simulink model "Bicycle_SCC_LKS"  (R2017a)
settings: Solver=ode45  StartTime=0.0  StopTime=30  MaxStep=0.001  RelTol=1e-3  EnableMultiTasking=on
PreLoadFcn:
  | load('Matrix.mat')
  | 
  | X0 = 25;         % 초기 X좌표 [m]
  | Y0 = 0;      % 초기 Y좌표 [m]
  | psi0 = 0;             % 초기 각도 [rad]
  | Vx0 = 100;           % 초기 속도 [km/h]
  | tf = 30;                 % 시뮬레이션 시간 [s]
  | 
  | % 제어기 설정 %
  | Q1 = 5;
  | Q2 = 3;
  | R =  2500;
  | PL = [-50-50i,-50+50i,-30,-20];
  | 
  | [K,L] = sfGain(Q1,Q2,R,PL);
model workspace (MAT data in the model file):
  Cf = 53220
  Cr = 39017
  Fx_Data = [-2029.26  -4058.51  -6087.76  -8117.01  -10146.3; -2029.26  -4058.51  -6087.76  -8117.01  -10146.3; -2053.55  -4107.12  -6160.67  -8214.24  -10267.8; -2084.58  -4169.16  -6253.75  -8338.33  -10422.9; -2125.47  -4250.95  -6376.42  -8501.91  -10627.4; -2181.64  -4363.28  -6544.93  -8726.56  -10908.2; -2262.94  -4525.87  -6788.82  -9051.76  -11314.7; -2388.22  -4776.46  -7164.69  -9552.92  -11941.1; -2476.95  -4953.9  -7430.85  -9907.79  -12384.7; -2586.89  -5173.78  -7760.68  -10347.6  -12934.4; -2634.75  -5269.5  -7904.24  -10539  -13173.7; -2680.7  -5361.4  -8042.1  -10722.8  -13403.5; -2717.36  -5434.73  -8152.09  -10869.4  -13586.8; -2729.82  -5459.63  -8189.45  -10919.3  -13649.1; -2689.78  -5379.54  -8069.32  -10759.1  -13448.8; -2548.95  -5097.92  -7646.88  -10195.8  -12744.8; -2240.07  -4480.13  -6720.21  -8960.27  -11200.3; -1701.43  -3402.86  -5104.29  -6805.72  -8507.15; -926.741  -1853.48  -2780.22  -3706.97  -4633.7; 0  0  0  0  0; 926.741  1853.48  2780.22  3706.97  4633.7; 1701.43  3402.86  5104.29  6805.72  8507.15; 2240.07  4480.13  6720.21  8960.27  11200.3; 2548.95  5097.92  7646.88  10195.8  12744.8; 2689.78  5379.54  8069.32  10759.1  13448.8; 2729.82  5459.63  8189.45  10919.3  13649.1; 2717.36  5434.73  8152.09  10869.4  13586.8; 2680.7  5361.4  8042.1  10722.8  13403.5; 2634.75  5269.5  7904.24  10539  13173.7; 2586.89  5173.78  7760.68  10347.6  12934.4; 2476.95  4953.9  7430.85  9907.79  12384.7; 2388.22  4776.46  7164.69  9552.92  11941.1; 2262.94  4525.87  6788.82  9051.76  11314.7; 2181.64  4363.28  6544.93  8726.56  10908.2; 2125.47  4250.95  6376.42  8501.91  10627.4; 2084.58  4169.16  6253.75  8338.33  10422.9; 2053.55  4107.12  6160.67  8214.24  10267.8; 2029.26  4058.51  6087.76  8117.01  10146.3; 2029.26  4058.51  6087.76  8117.01  10146.3]
  Fx_SL = [-1; -0.9; -0.8; -0.7; -0.6; -0.5; -0.4; -0.3; -0.25; -0.2; -0.18; -0.16; -0.14; -0.12; -0.1; -0.08; -0.06; -0.04; -0.02; 0; 0.02; 0.04; 0.06; 0.08; 0.1; 0.12; 0.14; 0.16; 0.18; 0.2; 0.25; 0.3; 0.4; 0.5; 0.6; 0.7; 0.8; 0.9; 1]
  Fx_W = [2105 3995 6120 7900 10100]
  Fy_Angle = [-20; -16; -14; -12; -10; -9.5; -9; -8.5; -8; -7.5; -7; -6.5; -6; -5.5; -5; -4.5; -4; -3.5; -3; -2.5; -2; -1.5; -1; -0.5; 0; 0.5; 1; 1.5; 2; 2.5; 3; 3.5; 4; 4.5; 5; 5.5; 6; 6.5; 7; 7.5; 8; 8.5; 9; 9.5; 10; 12; 14; 16; 18; 20]
  Fy_Data = [-1523.64 -1531.91 -1546.58 -1574.53 -1631.62 -1653.27 -1678.67 -1707.8 -1740.18 -1775.12 -1810.95 -1845.3 ... (250 elements, 50x5)]
  Fy_W = [1725 3500 6100 6950 9005]
  GearRatio = 17.25
  Iyy_Tire = 0.9
  Izz = 4192
  Pb2Tq_f = 300
  Pb2Tq_r = 150
  R_Tire = 0.33
  g = 9.81
  lf = 1.11
  lr = 1.6662
  m = 1530
  t2e = 2000
values from neighbouring files (symbols this model uses):
  P = polyfit(X*Scale,Y*Scale,4)    [Path_plot.m]
undefined symbols (not defined in the file or in its folder): A, B, K, L, sigbuilder_block
libraries: simulink x3
settings Model: Creator=Park  LastModifiedBy=edward
settings DataIOCC: SaveFormat=Array  SignalLoggingSaveFormat=ModelDataLogs
settings OptimizationCC: ExpressionDepthLimit=2147483647  LifeSpan=inf
settings DebuggingCC: UnderspecifiedInitializationDetection=Classic  MergeDetectMultiDrivingBlocksExec=none  SolverPrmCheckMsg=warning  MultiTaskDSMMsg=warning  MultiTaskCondExecSysMsg=none  FcnCallInpInsideContextMsg=warning  StateNameClashWarn=warning  StrictBusMsg=None  SFUnexpectedBacktrackingDiag=warning  SFNoUnconditionalDefaultTransitionDiag=warning  SFExecutionAtInitializationDiag=none
settings HardwareCC: ProdBitPerPointer=32  ProdBitPerSizeT=32  ProdBitPerPtrDiffT=32  ProdLargestAtomicFloat=None  ProdIntDivRoundTo=Undefined  ProdEndianess=Unspecified  ProdWordSize=32  ProdHWDeviceType=32-bit Generic
settings ModelReferenceCC: PropagateSignalLabelsOutOfModel=off
settings GRTTargetCC: TargetLangStandard=C89/C90 (ANSI)  GeneratePreprocessorConditionals=Disable all  CombineOutputUpdateFcns=off  GRTInterface=on
settings ConfigComp: CovMetricSettings=dw  CovHtmlReporting=on  CovSaveCumulativeToWorkspaceVar=on  CovSaveSingleToWorkspaceVar=on  CovExternalEMLEnable=off

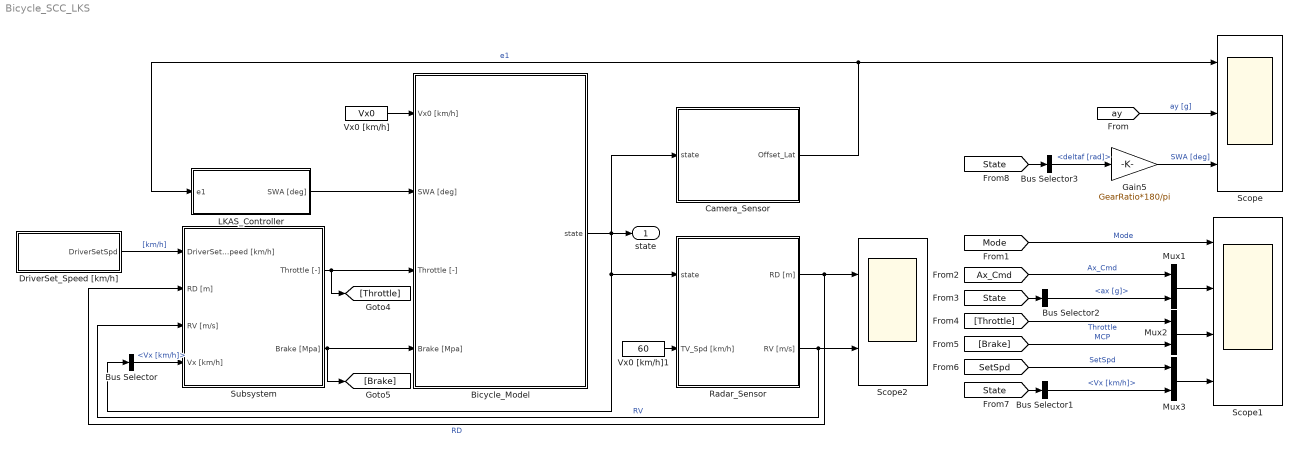
== system Bicycle_SCC_LKS ==
  Bicycle_Model : Subsystem
  Bus Selector : BusSelector  OutputSignals=Vx [km/h]
  Bus Selector1 : BusSelector  OutputSignals=Vx [km/h]
  Bus Selector2 : BusSelector  OutputSignals=ax [g]
  Bus Selector3 : BusSelector  OutputSignals=deltaf [rad]
  Camera_Sensor : Subsystem  TreatAsAtomicUnit=on  SystemSampleTime=1/100
  DriverSet_Speed [km/h] : Subsystem  Tag=STV Subsys  LoadFcn=sigbuilder_block('load');  StartFcn=sigbuilder_block('start');  StopFcn=sigbuilder_block('stop');  ClipboardFcn=sigbuilder_block('clipboard');  mask(Sigbuilder block){tuvar=[0:10]}
      mask help: Simulink:masks:SigbuilderBlock_MD
      mask init:
      | if ~strcmp(get_param(bdroot(gcbh),'SimulationStatus'),'stopped') tuvar = sigbuilder_block('maskInit'); end
      settings: CopyFcn=sigbuilder_block('copy');  DeleteFcn=sigbuilder_block('delete');  ModelCloseFcn=sigbuilder_block('modelClose');  PreSaveFcn=sigbuilder_block('preSave');  PauseFcn=sigbuilder_block('pause');  ContinueFcn=sigbuilder_block('continue');  NameChangeFcn=sigbuilder_block('namechange');  OpenFcn=sigbuilder_block('open',[6 36 708 710.25 ]);  CloseFcn=sigbuilder_block('close');
      mask Display: plot(0, 0, 100, 100,[2, 2, 32, 32, 2], [68, 8, 8, 68, 68],[32, 2], [38, 38], [32, 19, 2],[53, 60, 44], [32, 17, 17, 2],[16, 16, 31, 31]);txt = getActiveGroup(gcbh);text(2, 100, txt,'verticalAlignment', 'top');
  Gain5 : Gain  Gain=GearRatio*180/pi
  LKAS_Controller : Subsystem
  Mux1 : Mux  Inputs=2
  Mux2 : Mux  Inputs=2
  Mux3 : Mux  Inputs=2
  Radar_Sensor : Subsystem  SystemSampleTime=1/100
  Scope : Scope  NumInputPorts=3
  Scope1 : Scope  NumInputPorts=4
  Scope2 : Scope  NumInputPorts=2
  Subsystem : Subsystem
  Vx0 [km/h] : Constant  Value=Vx0
  Vx0 [km/h]1 : Constant  Value=60
  state : Outport
  wires:
  Vx0 [km/h]/1 -> Bicycle_Model/1(Vx0 [km/h])
  [ay] -> Scope/2  "ay [g]"
  Gain5/1 -> Scope/3  "SWA [deg]"
  DriverSet_Speed [km/h]/1(DriverSetSpd) -> Subsystem/1(DriverSet_Speed [km/h])  "[km/h]"
  [Mode] -> Scope1/1  "Mode"
  Mux1/1 -> Scope1/2
  [Ax_Cmd] -> Mux1/1  "Ax_Cmd"
  [State] -> Bus Selector2/1
  Mux2/1 -> Scope1/3
  [Brake] -> Mux2/2  "MCP"
  [Throttle] -> Mux2/1  "Throttle"
  Mux3/1 -> Scope1/4
  [SetSpd] -> Mux3/1  "SetSpd"
  LKAS_Controller/1(SWA [deg]) -> Bicycle_Model/2(SWA [deg])
  Bicycle_Model/1(state) -> Camera_Sensor/1(state), state/1, Radar_Sensor/1(state), Bus Selector/1
  Camera_Sensor/1(Offset_Lat) -> LKAS_Controller/1(e1), Scope/1  "e1"
  Subsystem/2(Brake [Mpa]) -> [Brake], Bicycle_Model/4(Brake [Mpa])
  Subsystem/1(Throttle [-]) -> Bicycle_Model/3(Throttle [-]), [Throttle]
  Bus Selector/1 -> Subsystem/4(Vx [km/h])  "<Vx [km/h]>"
  Radar_Sensor/1(RD [m]) -> Scope2/1, Subsystem/2(RD [m])  "RD"
  Radar_Sensor/2(RV [m/s]) -> Subsystem/3(RV [m/s]), Scope2/2  "RV"
  Vx0 [km/h]1/1 -> Radar_Sensor/2(TV_Spd [km/h])
  [State] -> Bus Selector1/1
  Bus Selector1/1 -> Mux3/2  "<Vx [km/h]>"
  Bus Selector2/1 -> Mux1/2  "<ax [g]>"
  [State] -> Bus Selector3/1
  Bus Selector3/1 -> Gain5/1  "<deltaf [rad]>"

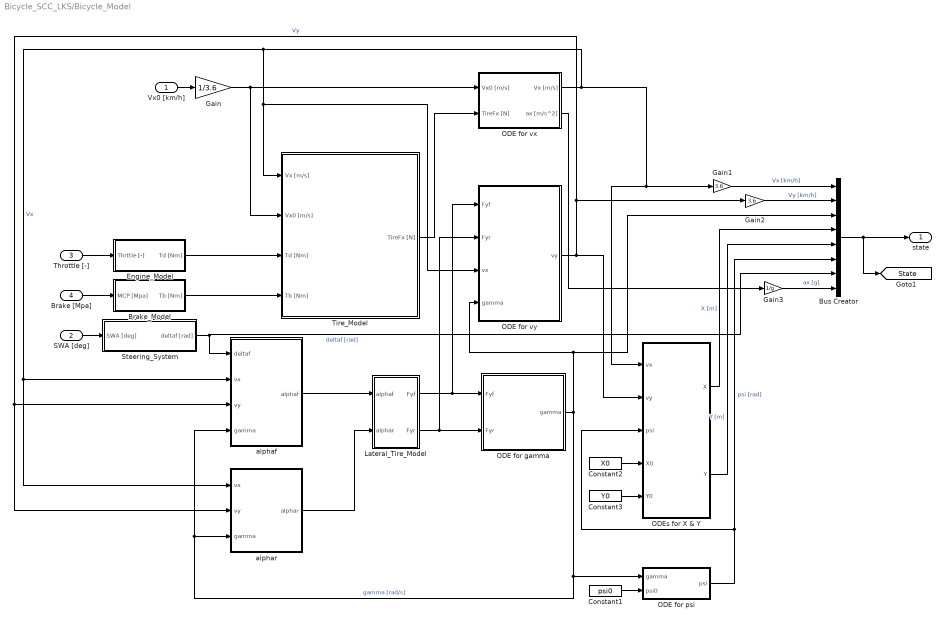
== system Bicycle_SCC_LKS/Bicycle_Model ==
  Vx0 [km/h] : Inport
  SWA [deg] : Inport  Port=2
  Throttle [-] : Inport  Port=3
  Brake [Mpa] : Inport  Port=4
  Brake_Model : Subsystem
  Bus Creator : BusCreator  Inputs=8
  Constant1 : Constant  Value=psi0
  Constant2 : Constant  Value=X0
  Constant3 : Constant  Value=Y0
  Engine_Model : Subsystem
  Gain : Gain  Gain=1/3.6
  Gain1 : Gain  Gain=3.6
  Gain2 : Gain  Gain=3.6
  Gain3 : Gain  Gain=1/g
  Lateral_Tire_Model : Subsystem
  ODE for gamma : Subsystem
  ODE for psi : Subsystem
  ODE for vx : Subsystem
  ODE for vy : Subsystem
  ODEs for X & Y : Subsystem
  Steering_System : Subsystem
  Tire_Model : Subsystem
  alphaf : Subsystem
  alphar : Subsystem
  state : Outport
  tag scope: State=global
  wires:
  alphaf/1(alphaf) -> Lateral_Tire_Model/1(alphaf)
  alphar/1(alphar) -> Lateral_Tire_Model/2(alphar)
  Lateral_Tire_Model/1(Fyf) -> ODE for vy/1(Fyf), ODE for gamma/1(Fyf)
  Lateral_Tire_Model/2(Fyr) -> ODE for vy/2(Fyr), ODE for gamma/2(Fyr)
  Bus Creator/1 -> [State], state/1
  Vx0 [km/h]/1 -> Gain/1
  Constant1/1 -> ODE for psi/2(psi0)
  SWA [deg]/1 -> Steering_System/1(SWA [deg])
  Constant2/1 -> ODEs for X & Y/4(X0)
  Constant3/1 -> ODEs for X & Y/5(Y0)
  ODE for psi/1(psi) -> ODEs for X & Y/3(psi), Bus Creator/6  "psi [rad]"
  ODEs for X & Y/1(X) -> Bus Creator/4  "X [m]"
  ODEs for X & Y/2(Y) -> Bus Creator/5  "Y [m]"
  Gain/1 -> ODE for vx/1(Vx0 [m/s]), Tire_Model/2(Vx0 [m/s])
  Engine_Model/1(Td [Nm]) -> Tire_Model/3(Td [Nm])
  Brake_Model/1(Tb [Nm]) -> Tire_Model/4(Tb [Nm])
  Brake [Mpa]/1 -> Brake_Model/1(MCP [Mpa])
  Throttle [-]/1 -> Engine_Model/1(Thrttle [-])
  Steering_System/1(deltaf [rad]) -> alphaf/1(deltaf), Bus Creator/7  "deltaf [rad]"
  ODE for vx/1(Vx [m/s]) -> alphaf/2(vx), alphar/1(vx), ODE for vy/3(vx), Tire_Model/1(Vx [m/s]), ODEs for X & Y/1(vx), Gain1/1  "Vx"
  ODE for gamma/1(gamma) -> Bus Creator/3, ODE for vy/4(gamma), ODE for psi/1(gamma), alphar/3(gamma), alphaf/4(gamma)  "gamma [rad/s]"
  Tire_Model/1(TireFx [N]) -> ODE for vx/2(TireFx [N])
  ODE for vx/2(ax [m/s^2]) -> Gain3/1
  ODE for vy/1(vy) -> alphar/2(vy), alphaf/3(vy), Gain2/1, ODEs for X & Y/2(vy)  "Vy"
  Gain1/1 -> Bus Creator/1  "Vx [km/h]"
  Gain2/1 -> Bus Creator/2  "Vy [km/h]"
  Gain3/1 -> Bus Creator/8  "ax [g]"

== system Bicycle_SCC_LKS/Camera_Sensor ==
  state : Inport
  Bus Selector : BusSelector  OutputSignals=X [m],Y [m],psi [rad]
  Compare To Constant : simulink/Logic and Bit Operations/Compare To Constant  relop=>=  const=350  OutDataTypeStr=boolean
  Gain : Gain  Gain=-1
  Level-2 MATLAB S-Function : M-S-Function  FunctionName=Error_Calculator_sfun
  Polynomial Coeff : Constant  Value=P
  Stop Simulation : Stop
  Terminator : Terminator
  Offset_Lat : Outport
  wires:
  state/1 -> Bus Selector/1
  Bus Selector/3 -> Level-2 MATLAB S-Function/4  "<psi [rad]>"
  Bus Selector/2 -> Level-2 MATLAB S-Function/3  "<Y [m]>"
  Bus Selector/1 -> Compare To Constant/1, Level-2 MATLAB S-Function/2  "<X [m]>"
  Level-2 MATLAB S-Function/1 -> Gain/1
  Polynomial Coeff/1 -> Level-2 MATLAB S-Function/1
  Level-2 MATLAB S-Function/2 -> Terminator/1
  Gain/1 -> Offset_Lat/1
  Compare To Constant/1 -> Stop Simulation/1

== system Bicycle_SCC_LKS/DriverSet_Speed [km//h] ==
  Demux : Demux  Tag=STV Demux  Outputs=1
  FromWs : FromWorkspace  Tag=STV FromWs  VariableName=tuvar  SampleTime=0
      SigBuilderData=|
      | common.afterFinalStr = 'Extrapolate'
      | common.sampleTime = 0
      | dataSet.timeRange = [0 30]
      | dataSet.name = 'Group 1'
      | sbobj.Groups.Name = 'Group 1'
      | sbobj.Groups.Signals.Name = 'DriverSetSpd'
      | sbobj.Groups.Signals.XData = [0 10 10 22 22 30]
      | sbobj.Groups.Signals.YData = [75 75 80 80 60 60]
      | sbobj.Groups.TimeRange = [0 30]
  DriverSetSpd : Outport  Tag=STV Outport
  wires:
  FromWs/1 -> Demux/1
  Demux/1 -> DriverSetSpd/1

== system Bicycle_SCC_LKS/LKAS_Controller ==
  e1 : Inport
  Ctrl_Law : Subsystem
  Observer : Subsystem
  Sum : Sum  Inputs=-+|
  SWA [deg] : Outport
  wires:
  Ctrl_Law/1(SWA [deg]) -> SWA [deg]/1, Observer/2(SWA [deg])
  Observer/1(e1_hat) -> Sum/1
  e1/1 -> Sum/2, Ctrl_Law/1(e1)
  Observer/2(e_hat) -> Ctrl_Law/2(e_hat)
  Sum/1 -> Observer/1(y_tilda)

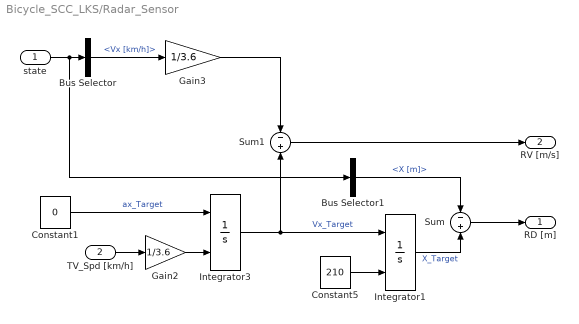
== system Bicycle_SCC_LKS/Radar_Sensor ==
  state : Inport
  TV_Spd [km/h] : Inport  Port=2
  Bus Selector : BusSelector  OutputSignals=Vx [km/h]
  Bus Selector1 : BusSelector  OutputSignals=X [m]
  Constant1 : Constant  Value=0
  Constant5 : Constant  Value=210
  Gain2 : Gain  Gain=1/3.6
  Gain3 : Gain  Gain=1/3.6
  Integrator1 : Integrator  InitialConditionSource=external  InitialCondition=500
  Integrator3 : Integrator  InitialConditionSource=external  InitialCondition=80  LimitOutput=on  LowerSaturationLimit=0
  Sum : Sum  Inputs=-+
  Sum1 : Sum  Inputs=-+
  RD [m] : Outport
  RV [m/s] : Outport  Port=2
  wires:
  TV_Spd [km/h]/1 -> Gain2/1
  Constant1/1 -> Integrator3/1  "ax_Target"
  Integrator3/1 -> Integrator1/1, Sum1/2  "Vx_Target"
  Integrator1/1 -> Sum/2  "X_Target"
  Constant5/1 -> Integrator1/2
  Sum/1 -> RD [m]/1
  Bus Selector1/1 -> Sum/1  "<X [m]>"
  Bus Selector/1 -> Gain3/1  "<Vx [km/h]>"
  Sum1/1 -> RV [m/s]/1
  Gain2/1 -> Integrator3/2
  Gain3/1 -> Sum1/1
  state/1 -> Bus Selector1/1, Bus Selector/1

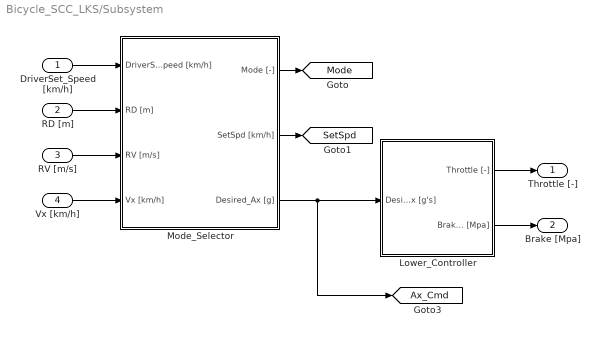
== system Bicycle_SCC_LKS/Subsystem ==
  DriverSet_Speed [km/h] : Inport
  RD [m] : Inport  Port=2
  RV [m/s] : Inport  Port=3
  Vx [km/h] : Inport  Port=4
  Lower_Controller : Subsystem
  Mode_Selector : Subsystem
  Throttle [-] : Outport
  Brake [Mpa] : Outport  Port=2
  tag scope: Ax_Cmd=global, Mode=global, SetSpd=global
  wires:
  Mode_Selector/3(Desired_Ax [g]) -> [Ax_Cmd], Lower_Controller/1(Desired_Ax [g's])
  Mode_Selector/1(Mode [-]) -> [Mode]
  Mode_Selector/2(SetSpd [km/h]) -> [SetSpd]
  RV [m/s]/1 -> Mode_Selector/3(RV [m/s])
  RD [m]/1 -> Mode_Selector/2(RD [m])
  DriverSet_Speed [km/h]/1 -> Mode_Selector/1(DriverSet_Speed [km/h])
  Vx [km/h]/1 -> Mode_Selector/4(Vx [km/h])
  Lower_Controller/1(Throttle [-]) -> Throttle [-]/1
  Lower_Controller/2(Brake [Mpa]) -> Brake [Mpa]/1

== system Bicycle_SCC_LKS/Bicycle_Model/Brake_Model ==
  MCP [Mpa] : Inport
  Gain : Gain  Gain=2*Pb2Tq_f
  Gain1 : Gain  Gain=2*Pb2Tq_r
  Mux : Mux  Inputs=2
  Transfer Fcn : TransferFcn  Denominator=[0.06 1]
  Transfer Fcn1 : TransferFcn  Denominator=[0.06 1]
  Tb [Nm] : Outport
  wires:
  Gain/1 -> Transfer Fcn/1  "Tb_f [Nm]"
  Gain1/1 -> Transfer Fcn1/1  "Tb_r [Nm]"
  MCP [Mpa]/1 -> Gain1/1, Gain/1
  Mux/1 -> Tb [Nm]/1
  Transfer Fcn/1 -> Mux/1
  Transfer Fcn1/1 -> Mux/2

== system Bicycle_SCC_LKS/Bicycle_Model/Engine_Model ==
  Thrttle [-] : Inport
  Gain : Gain  Gain=t2e
  Transfer Fcn : TransferFcn  Numerator=[100]  Denominator=[1 2*0.5*10 100]
  Td [Nm] : Outport
  wires:
  Thrttle [-]/1 -> Gain/1
  Gain/1 -> Transfer Fcn/1
  Transfer Fcn/1 -> Td [Nm]/1

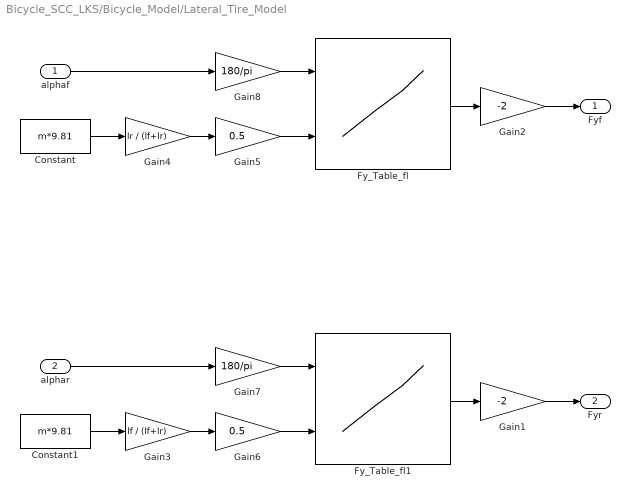
== system Bicycle_SCC_LKS/Bicycle_Model/Lateral_Tire_Model ==
  alphaf : Inport
  alphar : Inport  Port=2
  Constant : Constant  Value=m*9.81
  Constant1 : Constant  Value=m*9.81
  Fy_Table_fl : Lookup2D  RowIndex=Fy_Angle  ColumnIndex=Fy_W  Table=Fy_Data  LookUpMeth=Interpolation-Use End Values  SaturateOnIntegerOverflow=on
  Fy_Table_fl1 : Lookup2D  RowIndex=Fy_Angle  ColumnIndex=Fy_W  Table=Fy_Data  LookUpMeth=Interpolation-Use End Values  SaturateOnIntegerOverflow=on
  Gain1 : Gain  Gain=-2
  Gain2 : Gain  Gain=-2
  Gain3 : Gain  Gain=lf / (lf+lr)
  Gain4 : Gain  Gain=lr / (lf+lr)
  Gain5 : Gain  Gain=0.5
  Gain6 : Gain  Gain=0.5
  Gain7 : Gain  Gain=180/pi
  Gain8 : Gain  Gain=180/pi
  Fyf : Outport
  Fyr : Outport  Port=2
  wires:
  alphaf/1 -> Gain8/1
  Constant/1 -> Gain4/1
  Gain4/1 -> Gain5/1
  Gain5/1 -> Fy_Table_fl/2
  Fy_Table_fl/1 -> Gain2/1
  Gain2/1 -> Fyf/1
  Gain8/1 -> Fy_Table_fl/1
  alphar/1 -> Gain7/1
  Gain3/1 -> Gain6/1
  Gain6/1 -> Fy_Table_fl1/2
  Fy_Table_fl1/1 -> Gain1/1
  Gain7/1 -> Fy_Table_fl1/1
  Constant1/1 -> Gain3/1
  Gain1/1 -> Fyr/1

== system Bicycle_SCC_LKS/Bicycle_Model/ODE for gamma ==
  Fyf : Inport
  Fyr : Inport  Port=2
  Gain4 : Gain  Gain=1/Izz
  Gain5 : Gain  Gain=lf
  Gain6 : Gain  Gain=lr
  Integrator2 : Integrator
  Sum2 : Sum  Inputs=+-
  gamma : Outport
  wires:
  Sum2/1 -> Gain4/1
  Gain4/1 -> Integrator2/1
  Gain5/1 -> Sum2/1
  Gain6/1 -> Sum2/2
  Fyf/1 -> Gain5/1
  Integrator2/1 -> gamma/1  "gamma"
  Fyr/1 -> Gain6/1

== system Bicycle_SCC_LKS/Bicycle_Model/ODE for psi ==
  gamma : Inport
  psi0 : Inport  Port=2
  Integrator : Integrator  InitialConditionSource=external
  psi : Outport
  wires:
  gamma/1 -> Integrator/1  "dpsi"
  Integrator/1 -> psi/1
  psi0/1 -> Integrator/2

== system Bicycle_SCC_LKS/Bicycle_Model/ODE for vx ==
  Vx0 [m/s] : Inport
  TireFx [N] : Inport  Port=2
  Demux : Demux  Outputs=2
  Gain : Gain  Gain=1/m
  Integrator : Integrator  InitialConditionSource=external
  Sum : Sum
  Vx [m/s] : Outport
  ax [m/s^2] : Outport  Port=2
  wires:
  Vx0 [m/s]/1 -> Integrator/2
  Integrator/1 -> Vx [m/s]/1
  Sum/1 -> Gain/1
  Gain/1 -> Integrator/1, ax [m/s^2]/1
  TireFx [N]/1 -> Demux/1
  Demux/1 -> Sum/1
  Demux/2 -> Sum/2

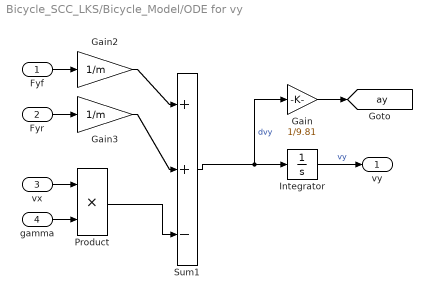
== system Bicycle_SCC_LKS/Bicycle_Model/ODE for vy ==
  Fyf : Inport
  Fyr : Inport  Port=2
  vx : Inport  Port=3
  gamma : Inport  Port=4
  Gain : Gain  Gain=1/9.81
  Gain2 : Gain  Gain=1/m
  Gain3 : Gain  Gain=1/m
  Integrator : Integrator
  Product : Product  RndMeth=Zero
  Sum1 : Sum  Inputs=++|-
  vy : Outport
  tag scope: ay=global
  wires:
  Gain2/1 -> Sum1/1
  Gain3/1 -> Sum1/2
  Sum1/1 -> Gain/1, Integrator/1  "dvy"
  Product/1 -> Sum1/3
  Fyf/1 -> Gain2/1
  Fyr/1 -> Gain3/1
  Integrator/1 -> vy/1  "vy"
  vx/1 -> Product/1
  gamma/1 -> Product/2
  Gain/1 -> [ay]

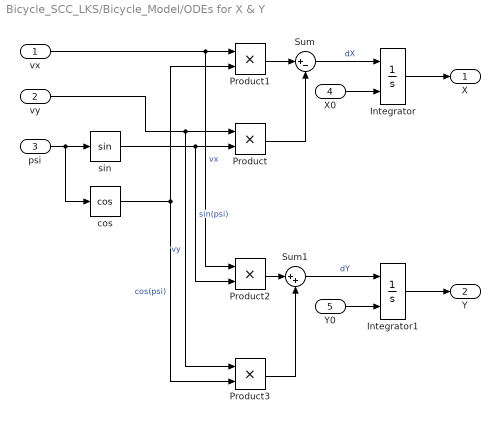
== system Bicycle_SCC_LKS/Bicycle_Model/ODEs for X & Y ==
  vx : Inport
  vy : Inport  Port=2
  psi : Inport  Port=3
  X0 : Inport  Port=4
  Y0 : Inport  Port=5
  Integrator : Integrator  InitialConditionSource=external  InitialCondition=42.14
  Integrator1 : Integrator  InitialConditionSource=external  InitialCondition=-0.3743
  Product{,1..3} (4 alike) : Product  RndMeth=Zero
  Sum : Sum  Inputs=|+-
  Sum1 : Sum  Inputs=|++
  cos : Trigonometry  Operator=cos
  sin : Trigonometry
  X : Outport
  Y : Outport  Port=2
  wires:
  psi/1 -> sin/1, cos/1
  sin/1 -> Product/2, Product2/2  "sin(psi)"
  vy/1 -> Product/1, Product3/1  "vy"
  vx/1 -> Product1/1, Product2/1  "vx"
  cos/1 -> Product1/2, Product3/2  "cos(psi)"
  Product1/1 -> Sum/1
  Product/1 -> Sum/2
  Sum/1 -> Integrator/1  "dX"
  Product2/1 -> Sum1/1
  Product3/1 -> Sum1/2
  Sum1/1 -> Integrator1/1  "dY"
  Integrator/1 -> X/1
  Integrator1/1 -> Y/1
  X0/1 -> Integrator/2
  Y0/1 -> Integrator1/2

== system Bicycle_SCC_LKS/Bicycle_Model/Steering_System ==
  SWA [deg] : Inport
  Gain : Gain  Gain=1/GearRatio
  Gain5 : Gain  Gain=pi/180
  Rate Limiter : RateLimiter  RisingSlewLimit=500  FallingSlewLimit=-500  SampleTimeMode=inherited
  Saturation : Saturate  UpperLimit=450  LowerLimit=-450
  deltaf [rad] : Outport
  wires:
  Gain/1 -> Gain5/1
  Gain5/1 -> deltaf [rad]/1
  SWA [deg]/1 -> Saturation/1
  Rate Limiter/1 -> Gain/1
  Saturation/1 -> Rate Limiter/1

== system Bicycle_SCC_LKS/Bicycle_Model/Tire_Model ==
  Vx [m/s] : Inport
  Vx0 [m/s] : Inport  Port=2
  Td [Nm] : Inport  Port=3
  Tb [Nm] : Inport  Port=4
  Long.Tire_Model : Subsystem
  ODE_for_Wss : Subsystem
  Slip_Ratio_Calculator : Subsystem
  TireFx [N] : Outport
  wires:
  Long.Tire_Model/1(TireFx [N]) -> TireFx [N]/1, ODE_for_Wss/1(TireFx [N])
  Slip_Ratio_Calculator/1(lamda [-]) -> Long.Tire_Model/1(lamda [-])
  Vx [m/s]/1 -> Slip_Ratio_Calculator/1(Vx [m/s])
  Vx0 [m/s]/1 -> ODE_for_Wss/2(Vx0 [m/s])
  Td [Nm]/1 -> ODE_for_Wss/3(Td [Nm])
  Tb [Nm]/1 -> ODE_for_Wss/4(Tb [Nm])
  ODE_for_Wss/1(Wss [rad/s]) -> Slip_Ratio_Calculator/2(Wss [rad/s])

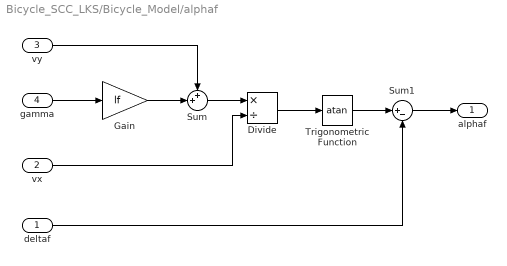
== system Bicycle_SCC_LKS/Bicycle_Model/alphaf ==
  deltaf : Inport
  vx : Inport  Port=2
  vy : Inport  Port=3
  gamma : Inport  Port=4
  Divide : Product  Inputs=*/
  Gain : Gain  Gain=lf
  Sum : Sum  Inputs=++|
  Sum1 : Sum  Inputs=|+-
  Trigonometric Function : Trigonometry  Operator=atan
  alphaf : Outport
  wires:
  gamma/1 -> Gain/1
  vy/1 -> Sum/1
  Gain/1 -> Sum/2
  Sum/1 -> Divide/1
  vx/1 -> Divide/2
  Divide/1 -> Trigonometric Function/1
  Trigonometric Function/1 -> Sum1/1
  deltaf/1 -> Sum1/2
  Sum1/1 -> alphaf/1

== system Bicycle_SCC_LKS/Bicycle_Model/alphar ==
  vx : Inport
  vy : Inport  Port=2
  gamma : Inport  Port=3
  Divide : Product  Inputs=*/
  Gain : Gain  Gain=lr
  Sum : Sum  Inputs=+-|
  Trigonometric Function : Trigonometry  Operator=atan
  alphar : Outport
  wires:
  Trigonometric Function/1 -> alphar/1
  Divide/1 -> Trigonometric Function/1
  vx/1 -> Divide/2
  Sum/1 -> Divide/1
  Gain/1 -> Sum/2
  vy/1 -> Sum/1
  gamma/1 -> Gain/1

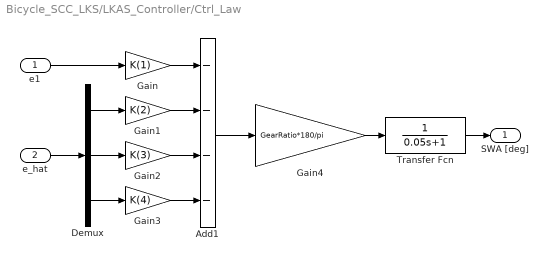
== system Bicycle_SCC_LKS/LKAS_Controller/Ctrl_Law ==
  e1 : Inport
  e_hat : Inport  Port=2
  Add1 : Sum  Inputs=----
  Demux : Demux  Outputs=3
  Gain : Gain  Gain=K(1)
  Gain1 : Gain  Gain=K(2)
  Gain2 : Gain  Gain=K(3)
  Gain3 : Gain  Gain=K(4)
  Gain4 : Gain  Gain=GearRatio*180/pi
  Transfer Fcn : TransferFcn  Denominator=[0.05 1]
  SWA [deg] : Outport
  wires:
  Gain3/1 -> Add1/4
  Gain2/1 -> Add1/3
  Gain1/1 -> Add1/2
  Demux/3 -> Gain3/1
  Demux/2 -> Gain2/1
  Demux/1 -> Gain1/1
  e1/1 -> Gain/1
  Gain/1 -> Add1/1
  e_hat/1 -> Demux/1
  Add1/1 -> Gain4/1
  Gain4/1 -> Transfer Fcn/1
  Transfer Fcn/1 -> SWA [deg]/1

== system Bicycle_SCC_LKS/LKAS_Controller/Observer ==
  y_tilda : Inport
  SWA [deg] : Inport  Port=2
  Demux : Demux
  Gain5 : Gain  Gain=1/GearRatio*pi/180
  Mux : Mux  Inputs=2
  Mux1 : Mux  Inputs=3
  State-Space : StateSpace  A=A  B=[B L']  C=diag([1 1 1 1])  D=zeros(4,2)  X0=0  ContinuousStateAttributes={'e1','e1_dot','e2','e2_dot'}
  e1_hat : Outport
  e_hat : Outport  Port=2
  wires:
  Mux/1 -> State-Space/1
  State-Space/1 -> Demux/1
  Demux/1 -> e1_hat/1  "e1_hat"
  y_tilda/1 -> Mux/2
  Demux/3 -> Mux1/2  "e2_hat"
  Demux/2 -> Mux1/1  "e1_dot_hat"
  Demux/4 -> Mux1/3  "e2_dot_hat"
  Mux1/1 -> e_hat/1
  SWA [deg]/1 -> Gain5/1
  Gain5/1 -> Mux/1

== system Bicycle_SCC_LKS/Subsystem/Lower_Controller ==
  Desired_Ax [g's] : Inport
  Brake_Controller : Subsystem  RequirementInfo={} %GIDa_b1ea8aed_7b1f_4164_abf5_d515769a3c42
  Throttle_Controller : Subsystem  RequirementInfo={} %GIDa_0f87ebad_d791_4b9c_99aa_9bea3fba617a
  Throttle [-] : Outport
  Brake [Mpa] : Outport  Port=2
  wires:
  Desired_Ax [g's]/1 -> Throttle_Controller/1(Ax_cmd [g's]), Brake_Controller/1(Ax_cmd [g's])
  Throttle_Controller/1(Throttle [-]) -> Throttle [-]/1
  Brake_Controller/1(Brake [Mpa]) -> Brake [Mpa]/1

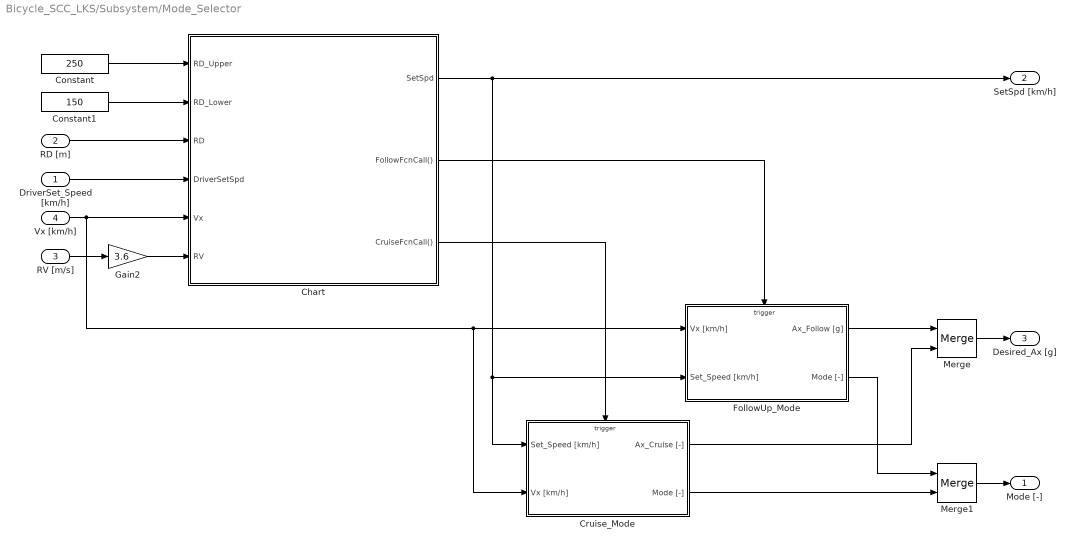
== system Bicycle_SCC_LKS/Subsystem/Mode_Selector ==
  DriverSet_Speed [km/h] : Inport
  RD [m] : Inport  Port=2
  RV [m/s] : Inport  Port=3
  Vx [km/h] : Inport  Port=4
  Chart : Stateflow chart  TreatAsAtomicUnit=on
  Constant : Constant  Value=250
  Constant1 : Constant  Value=150
  Cruise_Mode : Subsystem
  FollowUp_Mode : Subsystem
  Gain2 : Gain  Gain=3.6
  Merge : Merge
  Merge1 : Merge
  Mode [-] : Outport
  SetSpd [km/h] : Outport  Port=2
  Desired_Ax [g] : Outport  Port=3
  wires:
  Constant1/1 -> Chart/2(RD_Lower)
  Constant/1 -> Chart/1(RD_Upper)
  RV [m/s]/1 -> Gain2/1
  Cruise_Mode/2(Mode [-]) -> Merge1/2
  FollowUp_Mode/2(Mode [-]) -> Merge1/1
  Cruise_Mode/1(Ax_Cruise [-]) -> Merge/2
  FollowUp_Mode/1(Ax_Follow [g]) -> Merge/1
  Chart/1(SetSpd) -> SetSpd [km/h]/1, FollowUp_Mode/2(Set_Speed [km/h]), Cruise_Mode/1(Set_Speed [km/h])
  DriverSet_Speed [km/h]/1 -> Chart/4(DriverSetSpd)
  Chart/3(CruiseFcnCall()) -> Cruise_Mode/Trigger
  Chart/2(FollowFcnCall()) -> FollowUp_Mode/Trigger
  RD [m]/1 -> Chart/3(RD)
  Merge1/1 -> Mode [-]/1
  Merge/1 -> Desired_Ax [g]/1
  Vx [km/h]/1 -> Chart/5(Vx), Cruise_Mode/2(Vx [km/h]), FollowUp_Mode/1(Vx [km/h])
  Gain2/1 -> Chart/6(RV)

== system Bicycle_SCC_LKS/Bicycle_Model/Tire_Model/Long.Tire_Model ==
  lamda [-] : Inport
  Demux : Demux  Outputs=2
  Fx_f_Calculator : Subsystem
  Fx_r_Calculator : Subsystem
  Mux : Mux  Inputs=2
  TireFx [N] : Outport
  wires:
  lamda [-]/1 -> Demux/1
  Demux/1 -> Fx_f_Calculator/1(lamda_f [-])
  Demux/2 -> Fx_r_Calculator/1(lamda_r [-])
  Fx_f_Calculator/1(TireFx _f [N]) -> Mux/1
  Fx_r_Calculator/1(TireFx _r [N]) -> Mux/2
  Mux/1 -> TireFx [N]/1

== system Bicycle_SCC_LKS/Bicycle_Model/Tire_Model/ODE_for_Wss ==
  TireFx [N] : Inport
  Vx0 [m/s] : Inport  Port=2
  Td [Nm] : Inport  Port=3
  Tb [Nm] : Inport  Port=4
  Demux : Demux  Outputs=2
  Demux1 : Demux  Outputs=2
  Mux : Mux  Inputs=2
  ODE_for_Wss_f : Subsystem
  ODE_for_Wss_r : Subsystem
  Wss [rad/s] : Outport
  wires:
  Demux1/1 -> ODE_for_Wss_f/3(TireFx _f [N])  "TireFx _f [N]"
  Td [Nm]/1 -> ODE_for_Wss_f/1(Td_f [Nm])
  Vx0 [m/s]/1 -> ODE_for_Wss_r/1(Vx0 [m/s]), ODE_for_Wss_f/2(Vx0 [m/s])
  Tb [Nm]/1 -> Demux/1
  Demux/1 -> ODE_for_Wss_f/4(Tb_f [Nm])
  Demux/2 -> ODE_for_Wss_r/3(Tb_r [Nm])
  TireFx [N]/1 -> Demux1/1
  Demux1/2 -> ODE_for_Wss_r/2(TireFx _r [N])  "TireFx _r [N]"
  ODE_for_Wss_f/1(Wss_f [rad/s]) -> Mux/1
  ODE_for_Wss_r/1(Wss_r [rad/s]) -> Mux/2
  Mux/1 -> Wss [rad/s]/1

== system Bicycle_SCC_LKS/Bicycle_Model/Tire_Model/Slip_Ratio_Calculator ==
  Vx [m/s] : Inport
  Wss [rad/s] : Inport  Port=2
  Demux : Demux  Outputs=2
  Mux : Mux  Inputs=2
  lamda_f_Calculator : Subsystem
  lamda_r_Calculator1 : Subsystem
  lamda [-] : Outport
  wires:
  Vx [m/s]/1 -> lamda_f_Calculator/2(Vx [m/s]), lamda_r_Calculator1/2(Vx [m/s])
  lamda_f_Calculator/1(lamda_f [-]) -> Mux/1  "lamda_f [-]"
  lamda_r_Calculator1/1(lamda_r [-]) -> Mux/2  "lamda_r [-]"
  Mux/1 -> lamda [-]/1
  Wss [rad/s]/1 -> Demux/1
  Demux/1 -> lamda_f_Calculator/1(Wss_f [rad/s])  "Wss_f [rad/s]"
  Demux/2 -> lamda_r_Calculator1/1(Wss_r [rad/s])  "Wss_r [rad/s]"

== system Bicycle_SCC_LKS/Subsystem/Lower_Controller/Brake_Controller ==
  Ax_cmd [g's] : Inport
  Compare To Zero : simulink/Logic and Bit Operations/Compare To Zero  relop=<=  OutDataTypeStr=boolean
  Data Type Conversion : DataTypeConversion  OutDataTypeStr=double
  Gain : Gain  Gain=-1
  Gain1 : Gain  Gain=0.05
  Gain2 : Gain  Gain=12
  Integrator : Integrator  ExternalReset=rising
  Saturation : Saturate  UpperLimit=4  LowerLimit=0
  Sum : Sum
  Brake [Mpa] : Outport
  wires:
  Gain/1 -> Gain2/1, Gain1/1, Compare To Zero/1
  Saturation/1 -> Brake [Mpa]/1
  Sum/1 -> Saturation/1
  Ax_cmd [g's]/1 -> Gain/1
  Gain2/1 -> Sum/1
  Compare To Zero/1 -> Data Type Conversion/1
  Integrator/1 -> Sum/2
  Gain1/1 -> Integrator/1
  Data Type Conversion/1 -> Integrator/2

== system Bicycle_SCC_LKS/Subsystem/Lower_Controller/Throttle_Controller ==
  Ax_cmd [g's] : Inport
  Compare To Zero : simulink/Logic and Bit Operations/Compare To Zero  relop=<=  OutDataTypeStr=boolean
  Data Type Conversion : DataTypeConversion  OutDataTypeStr=double
  Gain1 : Gain  Gain=0.5
  Gain2 : Gain  Gain=7
  Integrator : Integrator  ExternalReset=rising
  Saturation : Saturate  UpperLimit=0.7  LowerLimit=0
  Sum : Sum
  Throttle [-] : Outport
  wires:
  Saturation/1 -> Throttle [-]/1
  Sum/1 -> Saturation/1
  Ax_cmd [g's]/1 -> Gain2/1, Gain1/1, Compare To Zero/1
  Gain2/1 -> Sum/1
  Compare To Zero/1 -> Data Type Conversion/1
  Integrator/1 -> Sum/2
  Gain1/1 -> Integrator/1
  Data Type Conversion/1 -> Integrator/2

== system Bicycle_SCC_LKS/Subsystem/Mode_Selector/Cruise_Mode ==
  Set_Speed [km/h] : Inport
  Vx [km/h] : Inport  Port=2
  function : TriggerPort  TriggerType=function-call  VariantControl=Variant
  Divide : Product  Inputs=/*
  Gain : Gain  Gain=1.2
  Mode1 : Constant  Value=0
  Saturation : Saturate  UpperLimit=0.3  LowerLimit=-0.3
  Sum : Sum  Inputs=|+-
  Ax_Cruise [-] : Outport
  Mode [-] : Outport  Port=2
  wires:
  Vx [km/h]/1 -> Sum/2
  Mode1/1 -> Mode [-]/1
  Saturation/1 -> Ax_Cruise [-]/1
  Divide/1 -> Gain/1  "Normalized_Vx"
  Sum/1 -> Divide/2
  Set_Speed [km/h]/1 -> Divide/1, Sum/1
  Gain/1 -> Saturation/1

== system Bicycle_SCC_LKS/Subsystem/Mode_Selector/FollowUp_Mode ==
  Vx [km/h] : Inport
  Set_Speed [km/h] : Inport  Port=2
  function : TriggerPort  TriggerType=function-call  VariantControl=Variant
  Divide : Product  Inputs=/*
  Gain : Gain  Gain=2
  Mode1 : Constant
  Saturation1 : Saturate  UpperLimit=0.4  LowerLimit=-0.4
  Sum1 : Sum  Inputs=|+-
  Ax_Follow [g] : Outport
  Mode [-] : Outport  Port=2
  wires:
  Vx [km/h]/1 -> Sum1/2
  Set_Speed [km/h]/1 -> Sum1/1, Divide/1
  Saturation1/1 -> Ax_Follow [g]/1
  Divide/1 -> Gain/1  "Normalized_Vx"
  Sum1/1 -> Divide/2
  Mode1/1 -> Mode [-]/1
  Gain/1 -> Saturation1/1

== system Bicycle_SCC_LKS/Bicycle_Model/Tire_Model/Long.Tire_Model/Fx_f_Calculator ==
  lamda_f [-] : Inport
  Constant : Constant  Value=m*9.81
  Fx_Table_fl : Lookup2D  RowIndex=Fx_SL  ColumnIndex=Fx_W  Table=Fx_Data  SaturateOnIntegerOverflow=on
  Gain : Gain  Gain=lr / (lf+lr)
  Gain1 : Gain  Gain=2
  Gain4 : Gain  Gain=0.5
  TireFx _f [N] : Outport
  wires:
  Gain1/1 -> TireFx _f [N]/1
  lamda_f [-]/1 -> Fx_Table_fl/1
  Constant/1 -> Gain/1
  Gain/1 -> Gain4/1
  Gain4/1 -> Fx_Table_fl/2  "Wf [N]"
  Fx_Table_fl/1 -> Gain1/1

== system Bicycle_SCC_LKS/Bicycle_Model/Tire_Model/Long.Tire_Model/Fx_r_Calculator ==
  lamda_r [-] : Inport
  Constant1 : Constant  Value=m*9.81
  Fx_Table_fl1 : Lookup2D  RowIndex=Fx_SL  ColumnIndex=Fx_W  Table=Fx_Data  SaturateOnIntegerOverflow=on
  Gain2 : Gain  Gain=lf / (lf+lr)
  Gain3 : Gain  Gain=2
  Gain5 : Gain  Gain=0.5
  TireFx _r [N] : Outport
  wires:
  lamda_r [-]/1 -> Fx_Table_fl1/1
  Constant1/1 -> Gain2/1
  Fx_Table_fl1/1 -> Gain3/1
  Gain2/1 -> Gain5/1
  Gain5/1 -> Fx_Table_fl1/2  "Wr [N]"
  Gain3/1 -> TireFx _r [N]/1

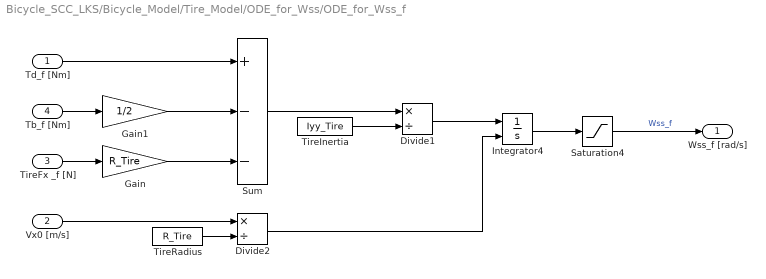
== system Bicycle_SCC_LKS/Bicycle_Model/Tire_Model/ODE_for_Wss/ODE_for_Wss_f ==
  Td_f [Nm] : Inport
  Vx0 [m/s] : Inport  Port=2
  TireFx _f [N] : Inport  Port=3
  Tb_f [Nm] : Inport  Port=4
  Divide1 : Product  Inputs=*/
  Divide2 : Product  Inputs=*/
  Gain : Gain  Gain=R_Tire
  Gain1 : Gain  Gain=1/2
  Integrator4 : Integrator  InitialConditionSource=external
  Saturation4 : Saturate  UpperLimit=255  LowerLimit=0
  Sum : Sum  Inputs=+--
  TireInertia : Constant  Value=Iyy_Tire
  TireRadius : Constant  Value=R_Tire
  Wss_f [rad/s] : Outport
  wires:
  Gain/1 -> Sum/3
  Td_f [Nm]/1 -> Sum/1
  Tb_f [Nm]/1 -> Gain1/1
  TireFx _f [N]/1 -> Gain/1
  Sum/1 -> Divide1/1
  TireInertia/1 -> Divide1/2
  Divide1/1 -> Integrator4/1
  TireRadius/1 -> Divide2/2
  Vx0 [m/s]/1 -> Divide2/1
  Divide2/1 -> Integrator4/2
  Integrator4/1 -> Saturation4/1
  Saturation4/1 -> Wss_f [rad/s]/1  "Wss_f"
  Gain1/1 -> Sum/2

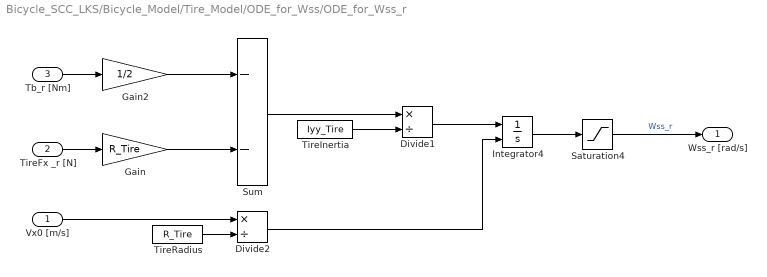
== system Bicycle_SCC_LKS/Bicycle_Model/Tire_Model/ODE_for_Wss/ODE_for_Wss_r ==
  Vx0 [m/s] : Inport
  TireFx _r [N] : Inport  Port=2
  Tb_r [Nm] : Inport  Port=3
  Divide1 : Product  Inputs=*/
  Divide2 : Product  Inputs=*/
  Gain : Gain  Gain=R_Tire
  Gain2 : Gain  Gain=1/2
  Integrator4 : Integrator  InitialConditionSource=external
  Saturation4 : Saturate  UpperLimit=255  LowerLimit=0
  Sum : Sum  Inputs=--
  TireInertia : Constant  Value=Iyy_Tire
  TireRadius : Constant  Value=R_Tire
  Wss_r [rad/s] : Outport
  wires:
  Saturation4/1 -> Wss_r [rad/s]/1  "Wss_r"
  Integrator4/1 -> Saturation4/1
  Divide2/1 -> Integrator4/2
  Vx0 [m/s]/1 -> Divide2/1
  TireRadius/1 -> Divide2/2
  Divide1/1 -> Integrator4/1
  TireInertia/1 -> Divide1/2
  Sum/1 -> Divide1/1
  TireFx _r [N]/1 -> Gain/1
  Tb_r [Nm]/1 -> Gain2/1
  Gain/1 -> Sum/2
  Gain2/1 -> Sum/1

== system Bicycle_SCC_LKS/Bicycle_Model/Tire_Model/Slip_Ratio_Calculator/lamda_f_Calculator ==
  Wss_f [rad/s] : Inport
  Vx [m/s] : Inport  Port=2
  Divide : Product  Inputs=*/
  Product2 : Product  RndMeth=Zero
  Saturation4 : Saturate  UpperLimit=1  LowerLimit=-1
  Subtract : Sum  Inputs=-+
  TireRadius : Constant  Value=R_Tire
  lamda_f [-] : Outport
  wires:
  Vx [m/s]/1 -> Subtract/1
  Wss_f [rad/s]/1 -> Product2/1
  TireRadius/1 -> Product2/2
  Product2/1 -> Subtract/2, Divide/2
  Subtract/1 -> Divide/1
  Divide/1 -> Saturation4/1
  Saturation4/1 -> lamda_f [-]/1

== system Bicycle_SCC_LKS/Bicycle_Model/Tire_Model/Slip_Ratio_Calculator/lamda_r_Calculator1 ==
  Wss_r [rad/s] : Inport
  Vx [m/s] : Inport  Port=2
  Divide : Product  Inputs=*/
  Product2 : Product  RndMeth=Zero
  Saturation4 : Saturate  UpperLimit=1  LowerLimit=-1
  Subtract : Sum  Inputs=-+
  TireRadius : Constant  Value=R_Tire
  lamda_r [-] : Outport
  wires:
  Saturation4/1 -> lamda_r [-]/1
  Divide/1 -> Saturation4/1
  Subtract/1 -> Divide/1
  Product2/1 -> Divide/2, Subtract/2
  TireRadius/1 -> Product2/2
  Wss_r [rad/s]/1 -> Product2/1
  Vx [m/s]/1 -> Subtract/1

== stateflow chart Bicycle_SCC_LKS/Subsystem/Mode_Selector/Chart ==
  state Cruise_Mode
    du, en : TVSpd = RV+Vx;
    du : send(CruiseFcnCall);
    du : SetSpd = DriverSetSpd;
  state FollowUp_Mode
    du, en : TVSpd = RV+Vx;
    du : send(FollowFcnCall);
    du : SetSpd = TVSpd;
  (default) -> Cruise_Mode
  Cruise_Mode -> FollowUp_Mode : [(RD <= RD_Lower) & (DriverSetSpd >= TVSpd)]
  FollowUp_Mode -> Cruise_Mode : [(RD >RD_Upper) | (DriverSetSpd < TVSpd)]
  data: RD_Upper input; RD_Lower input; RD input; DriverSetSpd input; SetSpd output; Vx input; RV input; TVSpd local
  events: FollowFcnCall output FUNCTION_CALL_EVENT; CruiseFcnCall output FUNCTION_CALL_EVENT
